simulink model "kinematic"  (R2016b)
settings: Solver=VariableStepAuto  StartTime=0.0  StopTime=80  RelTol=1e-3
values from neighbouring files (symbols this model uses):
  a = 0.18    [lqgfin.m]
  A = [-Ra1/La1     0            -Kb1/(r*La1)          -Kb1*l/(2*r*La1) ... (first row only)    [lqgfin.m]
  B = [1/La1 0 ... (first row only)    [lqgfin.m]
  C = [0    0    1/r  l/(2*r) ... (first row only)    [lqgfin.m]
  Cx = [0 0 1 0 0 0;0 0 0 1 0 0;0 0 0 0 1 0; 0 0 0 0 0 1]    [lqgfin.m]
  Cy = [1 0 0 0 0 0;0 1 0 0 0 0]    [lqgfin.m]
  kx = 0.1    [lqgfin.m]
  ky = 0.1    [lqgfin.m]
  l = 0.21    [lqgfin.m]
  ly = 0.1    [lqgfin.m]
  r = 0.13/2    (= 0.065)    [lqgfin.m]
undefined symbols (not defined in the file or in its folder): An, Bn, Cn, Dn, dumax, dwmax, K_lqi, umax, wmax
libraries: simulink x3, Controllers x2, DiffSteer_model x1
settings Model: Creator=Hamza  LastModifiedBy=Hamza

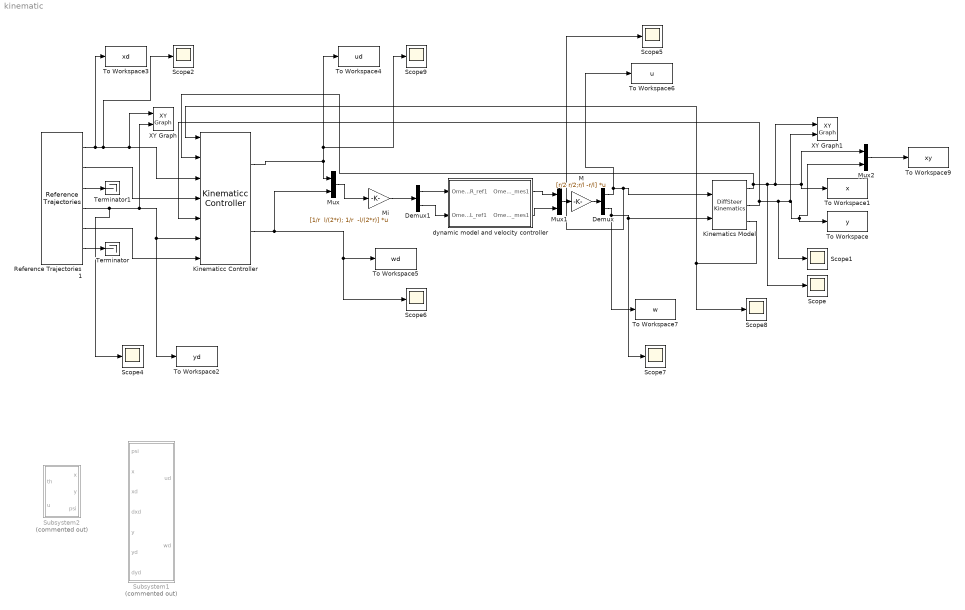
== system kinematic ==
  " Kinematics Model" : DiffSteer_model/DiffSteer Kinematics  x0=[0, 0, 0]  a=0.18  umax=1.3  wmax=12  dumax=5  dwmax=5
  Demux : Demux  Outputs=2
  Demux1 : Demux  Outputs=2
  Kinematicc Controller : Controllers/Kinematicc Controller  kx=1  ky=1  lx=0.25  ly=0.25  a=0
      link override 1//a: Gain=1/0.18
  M : Gain  Gain=[r/2 r/2;r/l -r/l]  Multiplication=Matrix(K*u)
  Mi : Gain  Gain="[1/r  l/(2*r); 1/r  -l/(2*r)]"  Multiplication=Matrix(K*u)
  Mux : Mux  Inputs=2
  Mux1 : Mux  Inputs=2
  Mux2 : Mux  Inputs=2
  Reference Trajectories1 : Controllers/Reference Trajectories  trajectory_type=2  wf=0.2  raio_ref_1=1  delta_raio=-0.2  t_delta_raio=100  xd=[2.5, 2.5]
  Scope{,1..2,4..9} (9 alike) : Scope
  Subsystem1 : Subsystem  Commented=on
  Subsystem2 : Subsystem  Commented=on
  Terminator : Terminator
  Terminator1 : Terminator
  To Workspace : ToWorkspace  VariableName=y  SampleTime=-1
  To Workspace1 : ToWorkspace  VariableName=x  SampleTime=-1
  To Workspace2 : ToWorkspace  VariableName=yd  SampleTime=-1
  To Workspace3 : ToWorkspace  VariableName=xd  SampleTime=-1
  To Workspace4 : ToWorkspace  VariableName=ud  SampleTime=-1
  To Workspace5 : ToWorkspace  VariableName=wd  SampleTime=-1
  To Workspace6 : ToWorkspace  VariableName=u  SampleTime=-1
  To Workspace7 : ToWorkspace  VariableName=w  SampleTime=-1
  To Workspace9 : ToWorkspace  VariableName=xy  SampleTime=-1
  XY Graph : simulink/Sinks/XY Graph  xmin=-10  xmax=10  ymin=-10  ymax=10  st=-1
  XY Graph1 : simulink/Sinks/XY Graph  xmin=-1.5  xmax=3  ymin=-1.5  ymax=3  st=-1
  dynamic model and velocity controller : Subsystem
  wires:
  Reference Trajectories1/1 -> Kinematicc Controller/3, XY Graph/1, Scope2/1, To Workspace3/1
  Reference Trajectories1/2 -> Kinematicc Controller/4
  Reference Trajectories1/4 -> Scope4/1, XY Graph/2, Kinematicc Controller/6, To Workspace2/1
  Reference Trajectories1/5 -> Kinematicc Controller/7
  " Kinematics Model"/1 -> Kinematicc Controller/2, Scope/1, XY Graph1/1, Mux2/1, To Workspace1/1
  " Kinematics Model"/2 -> Kinematicc Controller/5, Scope1/1, XY Graph1/2, Mux2/2, To Workspace/1
  " Kinematics Model"/3 -> Kinematicc Controller/1, Scope8/1
  Demux/2 -> " Kinematics Model"/2, Scope7/1, To Workspace7/1
  Reference Trajectories1/3 -> Terminator1/1
  Reference Trajectories1/6 -> Terminator/1
  Mux1/1 -> M/1
  Mux/1 -> Mi/1
  M/1 -> Demux/1
  Mi/1 -> Demux1/1
  Demux1/1 -> dynamic model and velocity controller/1(OmegaR_ref1)
  Demux1/2 -> dynamic model and velocity controller/2(OmegaL_ref1)
  dynamic model and velocity controller/1(OmegaR_mes1) -> Mux1/1
  dynamic model and velocity controller/2(OmegaL_mes1) -> Mux1/2
  Demux/1 -> " Kinematics Model"/1, Scope5/1, To Workspace6/1
  Mux2/1 -> To Workspace9/1
  Kinematicc Controller/1 -> Scope9/1, To Workspace4/1, Mux/1
  Kinematicc Controller/2 -> Scope6/1, To Workspace5/1, Mux/2

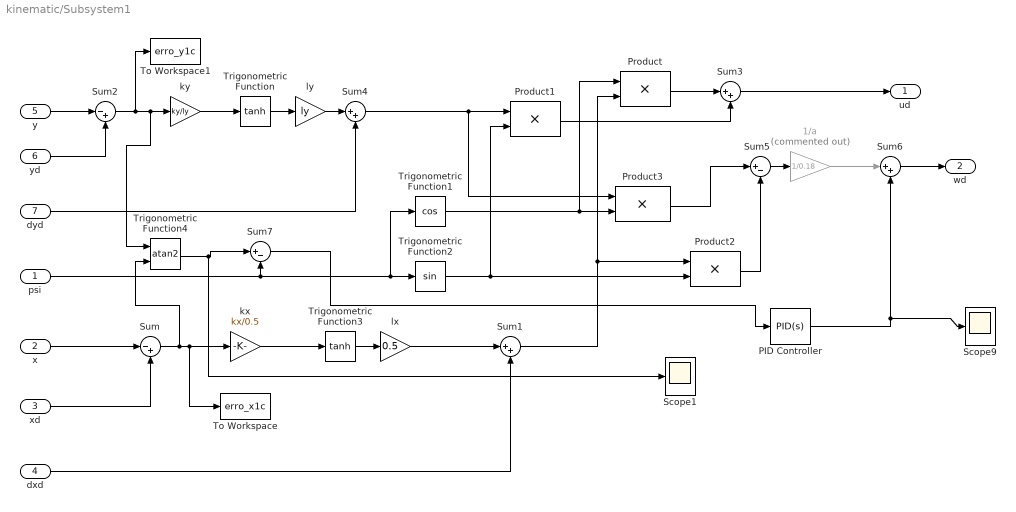
== system kinematic/Subsystem1 ==
  psi : Inport
  x : Inport  Port=2
  xd : Inport  Port=3
  dxd : Inport  Port=4
  y : Inport  Port=5
  yd : Inport  Port=6
  dyd : Inport  Port=7
  1/a : Gain  Commented=on  Gain=1/0.18  SaturateOnIntegerOverflow=on  OutDataTypeStr=Inherit: Same as input  ParamDataTypeStr=Inherit: Same as input
  PID Controller : simulink/Continuous/PID Controller  Controller=PID  TimeDomain=Continuous-time  SampleTime=-1  IntegratorMethod=Forward Euler  FilterMethod=Forward Euler  Form=Parallel  UseFilter=on  ControllerParametersSource=internal  P=10  I=1  D=0.5  N=100  InitialConditionSource=internal  InitialConditionForIntegrator=0  InitialConditionForFilter=0  ExternalReset=none  LimitOutput=off  UpperSaturationLimit=inf  LowerSaturationLimit=-inf  LinearizeAsGain=on  AntiWindupMode=none  Kb=1  TrackingMode=off  Kt=1  PParamMin=[]  PParamMax=[]  IParamMin=[]  IParamMax=[]  DParamMin=[]  DParamMax=[]  NParamMin=[]  NParamMax=[]  KbParamMin=[]  KbParamMax=[]  KtParamMin=[]  KtParamMax=[]  POutMin=[]  POutMax=[]  IOutMin=[]  IOutMax=[]  DOutMin=[]  DOutMax=[]  NOutMin=[]  NOutMax=[]  KbOutMin=[]  KbOutMax=[]  KtOutMin=[]  KtOutMax=[]  IntegratorOutMin=[]  IntegratorOutMax=[]  FilterOutMin=[]  FilterOutMax=[]  SumOutMin=[]  SumOutMax=[]  SumI1OutMin=[]  SumI1OutMax=[]  SumI2OutMin=[]  SumI2OutMax=[]  SumI3OutMin=[]  SumI3OutMax=[]  SumDOutMin=[]  SumDOutMax=[]  SaturationOutMin=[]  SaturationOutMax=[]  IntegratorContinuousStateAttributes=''  IntegratorStateMustResolveToSignalObject=off  IntegratorRTWStateStorageClass=Auto  FilterContinuousStateAttributes=''  FilterStateMustResolveToSignalObject=off  FilterRTWStateStorageClass=Auto  DifferentiatorICPrevScaledInput=0  DifferentiatorOutMin=[]  DifferentiatorOutMax=[]
  Product{,1..3} (4 alike) : Product  SaturateOnIntegerOverflow=on  OutDataTypeStr=Inherit: Same as first input
  Scope1 : Scope
  Scope9 : Scope
  Sum : Sum  Inputs=|-+  SaturateOnIntegerOverflow=on
  Sum{1,3..4,6} (4 alike) : Sum  Inputs=|++  SaturateOnIntegerOverflow=on
  Sum2 : Sum  Inputs=|-+  SaturateOnIntegerOverflow=on
  Sum5 : Sum  Inputs=|+-  SaturateOnIntegerOverflow=on
  Sum7 : Sum  Inputs=|+-  SaturateOnIntegerOverflow=on
  To Workspace : ToWorkspace  VariableName=erro_x1c  SampleTime=-1
  To Workspace1 : ToWorkspace  VariableName=erro_y1c  SampleTime=-1
  Trigonometric Function : Trigonometry  Operator=tanh
  Trigonometric Function1 : Trigonometry  Operator=cos
  Trigonometric Function2 : Trigonometry
  Trigonometric Function3 : Trigonometry  Operator=tanh
  Trigonometric Function4 : Trigonometry  Operator=atan2
  kx : Gain  Gain=kx/0.5  SaturateOnIntegerOverflow=on  OutDataTypeStr=Inherit: Same as input  ParamDataTypeStr=Inherit: Same as input
  ky : Gain  Gain=ky/ly  SaturateOnIntegerOverflow=on  OutDataTypeStr=Inherit: Same as input  ParamDataTypeStr=Inherit: Same as input
  lx : Gain  Gain=0.5  SaturateOnIntegerOverflow=on  OutDataTypeStr=Inherit: Same as input  ParamDataTypeStr=Inherit: Same as input
  ly : Gain  Gain=ly  SaturateOnIntegerOverflow=on  OutDataTypeStr=Inherit: Same as input  ParamDataTypeStr=Inherit: Same as input
  ud : Outport
  wd : Outport  Port=2
  wires:
  Sum7/1 -> PID Controller/1
  Trigonometric Function4/1 -> Sum7/1, Scope1/1
  PID Controller/1 -> Sum6/2, Scope9/1
  Sum6/1 -> wd/1
  1/a/1 -> Sum6/1
  Sum5/1 -> 1/a/1
  Trigonometric Function3/1 -> lx/1
  lx/1 -> Sum1/1
  Trigonometric Function/1 -> ly/1
  dyd/1 -> Sum4/2
  dxd/1 -> Sum1/2
  ly/1 -> Sum4/1
  Sum3/1 -> ud/1
  Product2/1 -> Sum5/2
  Product/1 -> Sum3/1
  Sum2/1 -> To Workspace1/1, ky/1, Trigonometric Function4/1
  Product3/1 -> Sum5/1
  Product1/1 -> Sum3/2
  Sum1/1 -> Product/2, Product2/1
  psi/1 -> Trigonometric Function1/1, Trigonometric Function2/1, Sum7/2
  x/1 -> Sum/1
  xd/1 -> Sum/2
  yd/1 -> Sum2/2
  Trigonometric Function1/1 -> Product/1, Product3/2
  kx/1 -> Trigonometric Function3/1
  ky/1 -> Trigonometric Function/1
  Trigonometric Function2/1 -> Product1/2, Product2/2
  Sum4/1 -> Product3/1, Product1/1
  y/1 -> Sum2/1
  Sum/1 -> To Workspace/1, kx/1, Trigonometric Function4/2

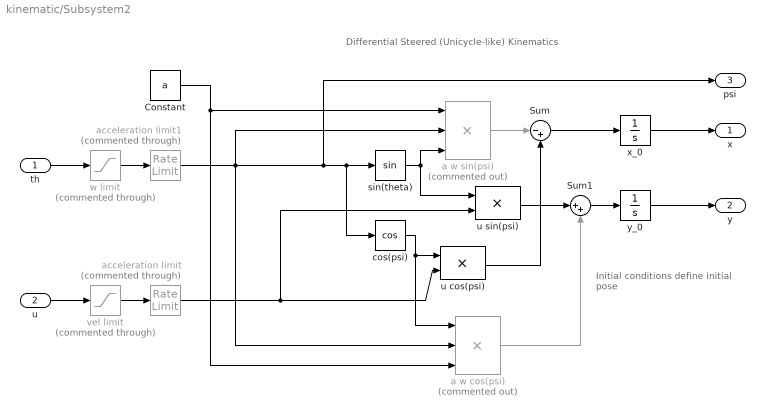
== system kinematic/Subsystem2 ==
  note: Initial conditions define
      | initial pose
  note: Differential Steered (Unicycle-like) Kinematics
  "th " : Inport
  u : Inport  Port=2
  Constant : Constant  Value=a
  Sum : Sum  Inputs=|-+  SaturateOnIntegerOverflow=on
  Sum1 : Sum  Inputs=|++  SaturateOnIntegerOverflow=on
  a w cos(psi) : Product  Commented=on  Inputs=3  SaturateOnIntegerOverflow=on  OutDataTypeStr=Inherit: Same as first input
  a w sin(psi) : Product  Commented=on  Inputs=3  SaturateOnIntegerOverflow=on  OutDataTypeStr=Inherit: Same as first input
  acceleration limit : RateLimiter  Commented=through  RisingSlewLimit=dumax  FallingSlewLimit=-dumax  SampleTimeMode=inherited
  acceleration limit1 : RateLimiter  Commented=through  RisingSlewLimit=dwmax  FallingSlewLimit=-dwmax  SampleTimeMode=inherited
  cos(psi) : Trigonometry  Operator=cos
  sin(theta) : Trigonometry
  u cos(psi) : Product  SaturateOnIntegerOverflow=on  OutDataTypeStr=Inherit: Same as first input
  u sin(psi) : Product  SaturateOnIntegerOverflow=on  OutDataTypeStr=Inherit: Same as first input
  vel limit : Saturate  Commented=through  UpperLimit=umax  LowerLimit=-umax
  w limit : Saturate  Commented=through  UpperLimit=wmax  LowerLimit=-wmax
  x_0 : Integrator
  y_0 : Integrator
  x : Outport
  y : Outport  Port=2
  psi : Outport  Port=3
  wires:
  x_0/1 -> x/1
  "th "/1 -> w limit/1
  u/1 -> vel limit/1
  Sum/1 -> x_0/1
  sin(theta)/1 -> a w sin(psi)/3, u sin(psi)/1
  a w cos(psi)/1 -> Sum1/2
  Constant/1 -> a w sin(psi)/1, a w cos(psi)/3
  u sin(psi)/1 -> Sum1/1
  w limit/1 -> acceleration limit1/1
  cos(psi)/1 -> u cos(psi)/1, a w cos(psi)/1
  u cos(psi)/1 -> Sum/2
  a w sin(psi)/1 -> Sum/1
  Sum1/1 -> y_0/1
  y_0/1 -> y/1
  acceleration limit/1 -> u sin(psi)/2, u cos(psi)/2
  acceleration limit1/1 -> sin(theta)/1, cos(psi)/1, psi/1, a w cos(psi)/2, a w sin(psi)/2
  vel limit/1 -> acceleration limit/1

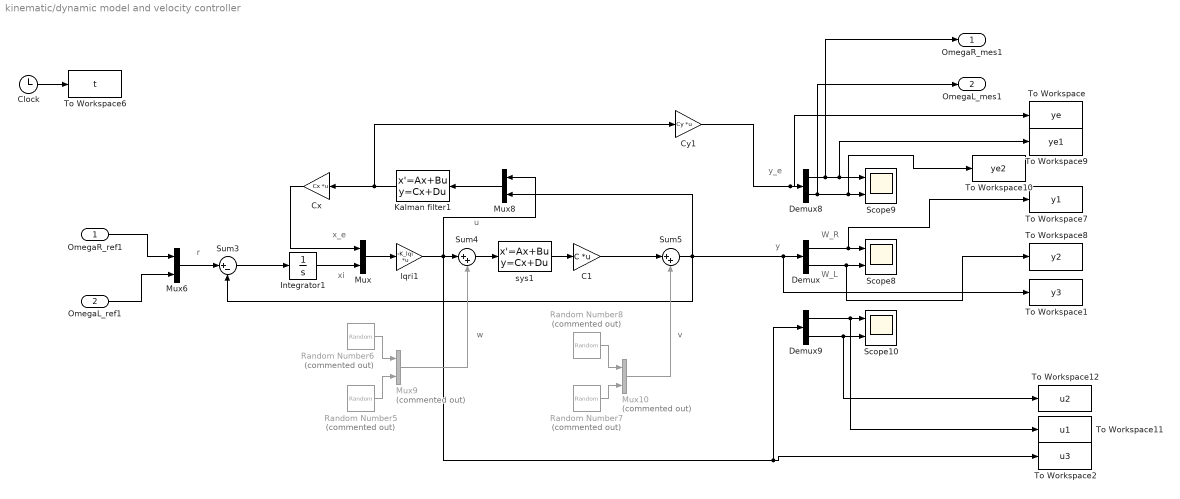
== system kinematic/dynamic model and velocity controller ==
  note: W_R
  note: r
  note: y_e
  note: xi
  note: x_e
  note: u
  note: y
  note: W_L
  note: w
  note: v
  OmegaR_ref1 : Inport
  OmegaL_ref1 : Inport  Port=2
  "  Cx" : Gain  Gain=Cx  Multiplication=Matrix(K*u)
  C1 : Gain  Gain=C  Multiplication=Matrix(K*u)
  Clock : Clock
  Cy1 : Gain  Gain=Cy  Multiplication=Matrix(K*u)
  Demux : Demux  Outputs=2
  Demux8 : Demux  Outputs=2
  Demux9 : Demux  Outputs=2
  Integrator1 : Integrator
  Kalman filter1 : StateSpace  A=An  B=Bn  C=Cn  D=Dn  X0=0
  Mux : Mux  Inputs=2
  Mux10 : Mux  Commented=on  Inputs=2
  Mux6 : Mux  Inputs=2
  Mux8 : Mux  Inputs=2
  Mux9 : Mux  Commented=on  Inputs=2
  Random Number5 : RandomNumber  Commented=on  Variance=0.1  Seed=40  SampleTime=0.01
  Random Number6 : RandomNumber  Commented=on  Variance=0.1  Seed=25  SampleTime=0.01
  Random Number7 : RandomNumber  Commented=on  Variance=0.1  Seed=30  SampleTime=0.01
  Random Number8 : RandomNumber  Commented=on  Variance=0.1  Seed=20  SampleTime=0.01
  Scope10 : Scope  NumInputPorts=2
  Scope8 : Scope  NumInputPorts=2
  Scope9 : Scope  NumInputPorts=2
  Sum3 : Sum  Inputs=|+-
  Sum4 : Sum  Inputs=|++
  Sum5 : Sum  Inputs=|++
  To Workspace : ToWorkspace  VariableName=ye  SampleTime=-1
  To Workspace1 : ToWorkspace  VariableName=y3  SampleTime=-1
  To Workspace10 : ToWorkspace  VariableName=ye2  SampleTime=-1
  To Workspace11 : ToWorkspace  VariableName=u1  SampleTime=-1
  To Workspace12 : ToWorkspace  VariableName=u2  SampleTime=-1
  To Workspace2 : ToWorkspace  VariableName=u3  SampleTime=-1
  To Workspace6 : ToWorkspace  VariableName=t  SampleTime=-1
  To Workspace7 : ToWorkspace  VariableName=y1  SampleTime=-1
  To Workspace8 : ToWorkspace  VariableName=y2  SampleTime=-1
  To Workspace9 : ToWorkspace  VariableName=ye1  SampleTime=-1
  lqri1 : Gain  Gain=-K_lqi  Multiplication=Matrix(K*u)
  sys1 : StateSpace  A=A  B=B  C=eye(4)  D=zeros(4,2)  X0=0
  OmegaR_mes1 : Outport
  OmegaL_mes1 : Outport  Port=2
  wires:
  Sum3/1 -> Integrator1/1
  Integrator1/1 -> Mux/2
  sys1/1 -> C1/1
  Mux/1 -> lqri1/1
  OmegaL_ref1/1 -> Mux6/2
  OmegaR_ref1/1 -> Mux6/1
  Mux6/1 -> Sum3/1
  Demux/1 -> To Workspace7/1, Scope8/1
  Demux/2 -> To Workspace8/1, Scope8/2
  Mux8/1 -> Kalman filter1/1
  Kalman filter1/1 -> Cy1/1, "  Cx"/1
  Random Number6/1 -> Mux9/1
  Random Number5/1 -> Mux9/2
  Random Number8/1 -> Mux10/1
  Random Number7/1 -> Mux10/2
  Sum5/1 -> Mux8/2, To Workspace1/1, Demux/1, Sum3/2
  Demux8/1 -> OmegaR_mes1/1, To Workspace9/1, Scope9/1
  Demux8/2 -> OmegaL_mes1/1, To Workspace10/1, Scope9/2
  Cy1/1 -> To Workspace/1, Demux8/1
  Sum4/1 -> sys1/1
  Demux9/1 -> To Workspace11/1, Scope10/1
  Demux9/2 -> To Workspace12/1, Scope10/2
  lqri1/1 -> Mux8/1, Demux9/1, To Workspace2/1, Sum4/1
  C1/1 -> Sum5/1
  Clock/1 -> To Workspace6/1
  Mux9/1 -> Sum4/2
  Mux10/1 -> Sum5/2
  "  Cx"/1 -> Mux/1
